simulink model "Controlador"  (R2022b)
settings: Solver=FixedStepAuto  StartTime=0.0  StopTime=inf  RelTol=1e-3  EnableMultiTasking=on
settings Model: ExtModeTrigDuration=2  Creator=dar.io  LastModifiedBy=dar.io
settings OptimizationCC: EnhancedBackFolding=on  PassReuseOutputArgsAs=Individual arguments  ZeroExternalMemoryAtStartup=off  ZeroInternalMemoryAtStartup=off  MaxStackSize=64  OptimizeBlockOrder=speed  DifferentSizesBufferReuse=on  OptimizationCustomize=off  EfficientTunableParamExpr=on
settings DebuggingCC: ParameterPrecisionLossMsg=none  ParameterTunabilityLossMsg=error
settings HardwareCC: ProdBitPerInt=16  ProdBitPerPointer=16  ProdBitPerSizeT=16  ProdBitPerPtrDiffT=16  ProdLargestAtomicFloat=None  ProdWordSize=8  ProdHWDeviceType=Atmel->AVR
settings SFSimCC: MATLABDynamicMemAlloc=off
settings RTWCC: Description=Embedded Coder  SystemTargetFile=ert.tlc  HardwareBoard=Arduino Mega 2560  TLCOptions=-aInlineSetEventsForThisBaseRateFcn=TLC_FALSE -aSuppressMultiTaskScheduler=TLC_FALSE -aRateBasedStepFcn=1  TemplateMakefile=ert_default_tmf  Toolchain=Arduino AVR  BuildConfiguration=Faster Runs
settings CodeAppCC: ForceParamTrailComments=on  IgnoreCustomStorageClasses=off  OperatorAnnotations=on  SimulinkDataObjDesc=on  SFDataObjDesc=on  InsertBlockDesc=on
settings ERTTargetCC: SupportContinuousTime=on  SupportVariableSizeSignals=on  ExtModeTransport=3  ExtModeStaticAlloc=on  ExtModeAutomaticAllocSize=off  ExtModeStaticAllocSize=2048  ExtModeMexFile=ext_xcp  ExtModeIntrfLevel=Level2 - Open

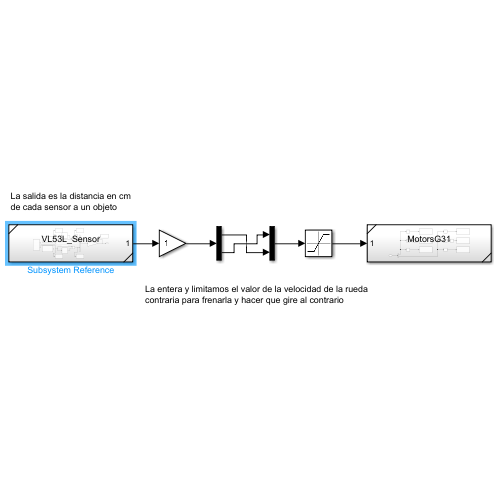
[thumbnail: Simulink's stored preview of the top-level diagram]
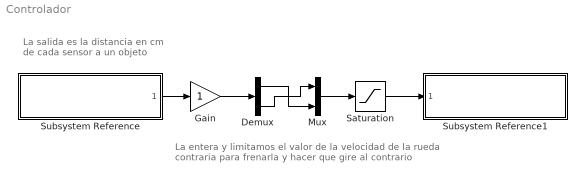
== system Controlador ==
  note: La entera y limitamos el valor de la velocidad de la rueda contraria para frenarla y hacer que gire al contrario
  note: La salida es la distancia en cm de cada sensor a un objeto
  Demux : Demux  Outputs=2
  Gain : Gain  OutDataTypeStr=int16
  Mux : Mux  Inputs=2
  Saturation : Saturate  UpperLimit=80  LowerLimit=0
  Subsystem Reference : Subsystem  ReferencedSubsystem=VL53L_Sensor
  Subsystem Reference1 : Subsystem  ReferencedSubsystem=MotorsG31
  wires:
  Subsystem Reference/1 -> Gain/1
  Saturation/1 -> Subsystem Reference1/1
  Mux/1 -> Saturation/1
  Demux/1 -> Mux/2
  Demux/2 -> Mux/1
  Gain/1 -> Demux/1
